simulink model "STEP7"  (R2020b)
settings: Solver=ode45  StartTime=0.0  StopTime=1400  RelTol=1e-3  EnableMultiTasking=on
settings Model: ExtModeTrigMode=oneshot  ExtModeArmWhenConnect=off  ExtModeAutoUpdateStatusClock=off  Creator=The MathWorks, Inc.  LastModifiedBy=Fong
settings SolverCC: InsertRTBMode=Auto
settings DataIOCC: SaveFormat=Array  SaveOutput=off  SaveTime=off  ReturnWorkspaceOutputs=off  SignalLoggingName=sigsOut
settings OptimizationCC: BlockReduction=off  BooleanDataType=off  ExpressionDepthLimit=2147483647  InitFltsAndDblsToZero=on  LifeSpan=1  EfficientTunableParamExpr=on
settings DebuggingCC: SaveWithParameterizedLinksMsg=none  UnderspecifiedInitializationDetection=Classic  MergeDetectMultiDrivingBlocksExec=none  SignalResolutionControl=TryResolveAllWithWarning  MultiTaskDSMMsg=warning  MultiTaskCondExecSysMsg=none  FcnCallInpInsideContextMsg=warning  StateNameClashWarn=warning  SFUnexpectedBacktrackingDiag=warning  SFNoUnconditionalDefaultTransitionDiag=warning  SFExecutionAtInitializationDiag=none  ArithmeticOperatorsInVariantConditions=warning
settings HardwareCC: ProdBitPerPointer=32  ProdBitPerSizeT=32  ProdBitPerPtrDiffT=32  ProdLargestAtomicFloat=None  ProdIntDivRoundTo=Undefined  ProdEndianess=Unspecified  ProdWordSize=32  ProdHWDeviceType=ASIC/FPGA  TargetUnknown=on  ProdEqTarget=off
settings ModelReferenceCC: PropagateSignalLabelsOutOfModel=off
settings SFSimCC: SFSimEcho=off  SimUseLocalCustomCode=off  SimParseCustomCode=off  CustomCodeUndefinedFunction=UseInterfaceOnly
settings RTWCC: SystemTargetFile=ert.tlc  GenCodeOnly=on  TemplateMakefile=ert_default_tmf  GenerateReport=on  RTWVerbose=off  RTWUseLocalCustomCode=off  IncludeHyperlinkInReport=on  LaunchReport=on
settings CodeAppCC: IgnoreCustomStorageClasses=off  CustomSymbolStrType=$N$R$M  CustomSymbolStrModelFcn=$N  StateflowObjectComments=on  InternalIdentifier=Classic
settings ERTTargetCC: TargetFcnLib=ansi_tfl_tmw.mat  MultiwordLength=2048  GenerateSampleERTMain=on  SupportContinuousTime=on  SupportNonInlinedSFcns=on  ERTCustomFileTemplate=example_file_process.tlc  ConvertIfToSwitch=off  SuppressUnreachableDefaultCases=off
settings ConfigComp: CovMetricSettings=dcmtr  CovSaveCumulativeToWorkspaceVar=on  CovSaveSingleToWorkspaceVar=on  CovExternalEMLEnable=off  CovSFcnEnable=off

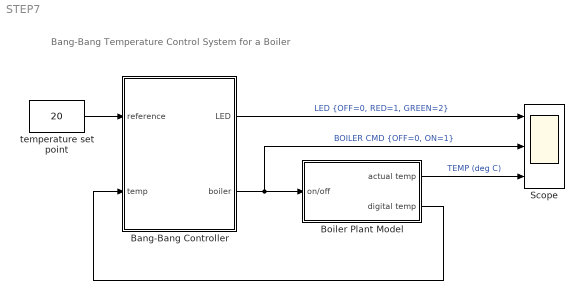
== system STEP7 ==
  note: Bang-Bang Temperature Control System for a Boiler
  Bang-Bang Controller : Stateflow chart  TreatAsAtomicUnit=on
  Boiler Plant Model : Subsystem
  Scope : Scope  NumInputPorts=3
  temperature set point : Constant  Value=20  OutDataTypeStr=Inherit: Inherit via back propagation
  wires:
  Bang-Bang Controller/2(" boiler") -> Scope/2, Boiler Plant Model/1(on/off)  "BOILER CMD {OFF=0, ON=1}"
  temperature set point/1 -> Bang-Bang Controller/1(reference)
  Boiler Plant Model/2(digital temp) -> Bang-Bang Controller/2(temp)
  Boiler Plant Model/1(actual temp) -> Scope/3  "TEMP (deg C)"
  Bang-Bang Controller/1(LED) -> Scope/1  "LED {OFF=0, RED=1, GREEN=2}"

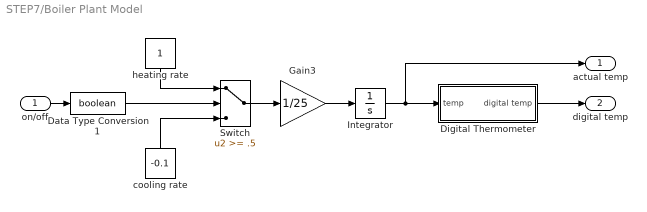
== system STEP7/Boiler Plant Model ==
  on/off : Inport
  Data Type Conversion1 : DataTypeConversion  OutDataTypeStr=boolean  SaturateOnIntegerOverflow=on  RndMeth=Zero
  Digital Thermometer : Subsystem
  Gain3 : Gain  Gain=1/25  SaturateOnIntegerOverflow=on  OutDataTypeStr=Inherit: Same as input  ParamDataTypeStr=Inherit: Same as input
  Integrator : Integrator  InitialCondition=15  ZeroCross=off
  Switch : Switch  Threshold=.5  SaturateOnIntegerOverflow=on  InputSameDT=on
  cooling rate : Constant  Value=-0.1
  heating rate : Constant
  actual temp : Outport  VectorParamsAs1DForOutWhenUnconnected=off
  digital temp : Outport  Port=2  VectorParamsAs1DForOutWhenUnconnected=off
  wires:
  Gain3/1 -> Integrator/1
  cooling rate/1 -> Switch/3
  heating rate/1 -> Switch/1
  Switch/1 -> Gain3/1
  on/off/1 -> Data Type Conversion1/1
  Data Type Conversion1/1 -> Switch/2
  Integrator/1 -> actual temp/1, Digital Thermometer/1(temp)
  Digital Thermometer/1(digital temp) -> digital temp/1

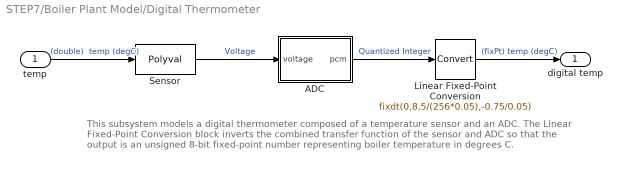
== system STEP7/Boiler Plant Model/Digital Thermometer ==
  note: This subsystem models a digital thermometer composed of a temperature sensor and an ADC.
      | The Linear Fixed-Point Conversion block inverts the combined transfer function of the sensor and ADC
      | so that the output is an unsigned 8-bit fixed-point number representing boiler temperature in degrees C.
  temp : Inport
  ADC : Subsystem
      mask Display: fprintf('ADC\n8-bit\n0-5V');
  Linear Fixed-Point Conversion : DataTypeConversion  OutDataTypeStr=fixdt(0,8,5/(256*0.05),-0.75/0.05)  ConvertRealWorld=Stored Integer (SI)
  Sensor : Polyval  Coefs="[ 0.05     0.75 ]"
  digital temp : Outport  VectorParamsAs1DForOutWhenUnconnected=off
  wires:
  temp/1 -> Sensor/1  "(double)  temp (degC)"
  Linear Fixed-Point Conversion/1 -> digital temp/1  "(fixPt) temp (degC)"
  Sensor/1 -> ADC/1(voltage)  "Voltage"
  ADC/1(pcm) -> Linear Fixed-Point Conversion/1  "Quantized Integer"

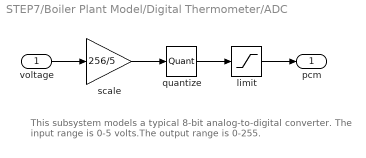
== system STEP7/Boiler Plant Model/Digital Thermometer/ADC ==
  note: This subsystem models a typical 8-bit analog-to-digital converter. The input range is 0-5 volts.The output range is 0-255.
  voltage : Inport
  limit : Saturate  UpperLimit=255  LowerLimit=0
  quantize : Quantizer  QuantizationInterval=1
  scale : Gain  Gain=256/5  SaturateOnIntegerOverflow=on  OutDataTypeStr=Inherit: Same as input  ParamDataTypeStr=Inherit: Same as input
  pcm : Outport  VectorParamsAs1DForOutWhenUnconnected=off
  wires:
  voltage/1 -> scale/1
  quantize/1 -> limit/1
  scale/1 -> quantize/1
  limit/1 -> pcm/1

== stateflow chart STEP7/Bang-Bang Controller ==
  settings: updateMethod=DISCRETE  sampleTime=1
  state Heater [group]
    state Off
      en: LED = RED;
      state Flash
        en: flash_LED()
      Flash -> Flash : after(5,sec)
    state On
      en,du: flash_LED()
      (history)
      state HIGH
      state NORM
      (default) -> HIGH
      HIGH -> NORM : [warm()]
    (default) -> Off
    On -> Off : after(20,sec)
    Off -> On : after(40,sec)[cold()]
    NORM -> Off : [warm()]
  state flash_LED [function]
    (default) -> (junction 60)
    (junction 60) -> (junction 62) [order 1] : [boiler == ON]
    (junction 60) -> (junction 66) [order 2] : {color=RED}
    (junction 62) -> (junction 64) : {color=GREEN}
    (junction 64) -> (junction 66)
    (junction 66) -> (junction 37)
    (junction 37) -> (junction 38) [order 1] : [LED == color]
    (junction 37) -> (junction 31) [order 2] : {LED=color}
    (junction 38) -> (junction 42) : {LED=OFF}
  state b = cold [function]
    (default) -> (junction 39) : { b = temp<=reference}
  state b = warm [function]
    (default) -> (junction 72) : {b = ~cold()}
  data: b function_output boolean; b function_output boolean; LED output int8; color local int8; reference input fixdt(0,8,1,-15); GREEN constant int8 =2; OFF constant int8 =0; ON constant int8 =1; RED constant int8 =1; temp input fixdt(0,8,5/(256*0.05),-0.75/0.05); boiler output boolean
